simulink model "fetft_transfer_function_block_diagram"  (R2026a)
settings: Solver=ode45  StopTime=8e-05  MaxStep=1e-07
settings Model: Creator=elesamj  LastModifiedBy=elesamj

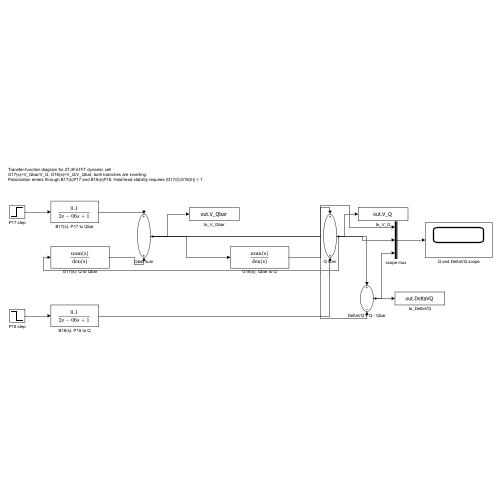
[thumbnail: Simulink's stored preview of the top-level diagram]
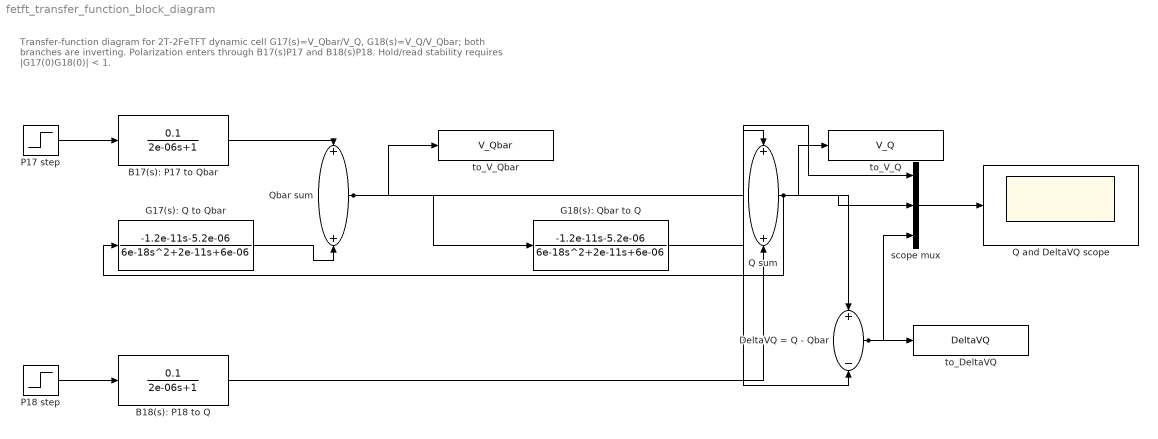
== system fetft_transfer_function_block_diagram ==
  note: Transfer-function diagram for 2T-2FeTFT dynamic cell
      | G17(s)=V_Qbar/V_Q, G18(s)=V_Q/V_Qbar; both branches are inverting.
      | Polarization enters through B17(s)P17 and B18(s)P18. Hold/read stability requires |G17(0)G18(0)| < 1.
  B17(s): P17 to Qbar : TransferFcn  Numerator=0.1  Denominator=[2e-06 1]
  B18(s): P18 to Q : TransferFcn  Numerator=0.1  Denominator=[2e-06 1]
  DeltaVQ = Q - Qbar : Sum  Inputs=+-
  G17(s): Q to Qbar : TransferFcn  Numerator=[-1.2e-11 -5.2e-06]  Denominator=[6e-18 2e-11 6e-06]
  G18(s): Qbar to Q : TransferFcn  Numerator=[-1.2e-11 -5.2e-06]  Denominator=[6e-18 2e-11 6e-06]
  P17 step : Step  Time=1e-06  FinalValue=0.5  SampleTime=0
  P18 step : Step  Time=1e-06  FinalValue=-0.5  SampleTime=0
  Q and DeltaVQ scope : Scope
  Q sum : Sum
  Qbar sum : Sum
  scope mux : Mux  Inputs=3
  to_DeltaVQ : ToWorkspace  VariableName=DeltaVQ  SaveFormat=Structure With Time  SampleTime=-1
  to_V_Q : ToWorkspace  VariableName=V_Q  SaveFormat=Structure With Time  SampleTime=-1
  to_V_Qbar : ToWorkspace  VariableName=V_Qbar  SaveFormat=Structure With Time  SampleTime=-1
  wires:
  P17 step/1 -> B17(s): P17 to Qbar/1
  B17(s): P17 to Qbar/1 -> Qbar sum/1
  Qbar sum/1 -> to_V_Qbar/1, G18(s): Qbar to Q/1, DeltaVQ = Q - Qbar/2, scope mux/1
  G18(s): Qbar to Q/1 -> Q sum/1
  P18 step/1 -> B18(s): P18 to Q/1
  B18(s): P18 to Q/1 -> Q sum/2
  Q sum/1 -> to_V_Q/1, G17(s): Q to Qbar/1, DeltaVQ = Q - Qbar/1, scope mux/2
  G17(s): Q to Qbar/1 -> Qbar sum/2
  DeltaVQ = Q - Qbar/1 -> to_DeltaVQ/1, scope mux/3
  scope mux/1 -> Q and DeltaVQ scope/1
